simulink model "l2p2q6d"  (R2020b)
settings: Solver=VariableStepAuto  StartTime=0.0  StopTime=10.0  RelTol=1e-3
values from neighbouring files (symbols this model uses):
  a0 = b/m_l    (= 273.076923077)    [l2p1q2.m]    (also in l2p1q3.m; l2p2q7.m)
  b0 = k/m_l    (= 273.076923077)    [l2p1q2.m]    (also in l2p2q7.m)
  b1 = d/m_l    (= 3.84615384615)    [l2p1q2.m]    (also in l2p1q3.m; l2p2q7.m)
  c0 = alpha*k    (= 215.3714)    [l2p2q7.m]
  c1 = alpha*d    (= 3.0334)    [l2p2q7.m]
  c2 = alpha*m_l    (= 0.788684)    [l2p2q7.m]
  d1 = k*(d+v-beta)    (= 2015.9314)    [l2p2q7.m]
  d2 = (m_l+m_m)*k + (v-beta)*d    (= 231.7134)    [l2p2q7.m]
  d3 = m_m*d + (v-beta)*m_l    (= 8.222284)    [l2p2q7.m]
  d4 = m_m*m_l    (= 0.4888)    [l2p2q7.m]
settings Model: Creator=thaibinhbr97  LastModifiedBy=thaibinhbr97

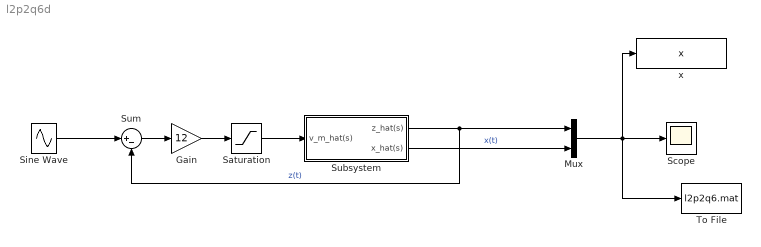
== system l2p2q6d ==
  Gain : Gain  Gain=12
  Mux : Mux  Inputs=2
  Saturation : Saturate  UpperLimit=2.5  LowerLimit=-2.5
  Scope : Scope
  Sine Wave : Sin  Amplitude=0.4  Frequency=16.5  SampleTime=0
  Subsystem : Subsystem
  Sum : Sum  Inputs=|+-
  To File : ToFile  Filename=l2p2q6.mat  SaveFormat=Timeseries
  x : ToWorkspace  VariableName=x  SaveFormat=Timeseries  SampleTime=-1
  wires:
  Subsystem/1(z_hat(s)) -> Mux/1, Sum/2  "z(t)"
  Subsystem/2(x_hat(s)) -> Mux/2  "x(t)"
  Mux/1 -> x/1, To File/1, Scope/1
  Sine Wave/1 -> Sum/1
  Saturation/1 -> Subsystem/1(v_m_hat(s))
  Gain/1 -> Saturation/1
  Sum/1 -> Gain/1

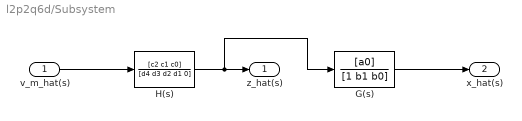
== system l2p2q6d/Subsystem ==
  v_m_hat(s) : Inport
  G(s) : TransferFcn  Numerator=[a0]  Denominator=[1 b1 b0]
  H(s) : TransferFcn  Numerator=[c2 c1 c0]  Denominator=[d4 d3 d2 d1 0]
  z_hat(s) : Outport
  x_hat(s) : Outport  Port=2
  wires:
  v_m_hat(s)/1 -> H(s)/1
  H(s)/1 -> G(s)/1, z_hat(s)/1
  G(s)/1 -> x_hat(s)/1
